simulink model "Feedback_2"  (R2017b)
settings: Solver=FixedStepDiscrete  StartTime=0.0  StopTime=10.0  FixedStep=.0001  RelTol=1e-3  EnableMultiTasking=on
libraries: stellaris_lp_lib x12, simulink x1
settings Model: Creator=Mitchell Cassaday  LastModifiedBy=Mitchell Cassaday
settings OptimizationCC: PassReuseOutputArgsAs=Individual arguments  MaxStackSize=64
settings DebuggingCC: ParameterTunabilityLossMsg=error
settings HardwareCC: ProdBitPerPointer=32  ProdBitPerSizeT=32  ProdBitPerPtrDiffT=32  ProdLargestAtomicInteger=Long  ProdLargestAtomicFloat=Double  ProdWordSize=32  ProdHWDeviceType=ARM Compatible->ARM Cortex
settings SFSimCC: MATLABDynamicMemAlloc=off
settings RTWCC: SystemTargetFile=ert.tlc  HardwareBoard=Tiva TM4C123G Launchpad  TLCOptions=-aInlineSetEventsForThisBaseRateFcn=TLC_FALSE -aSuppressMultiTaskScheduler=TLC_FALSE -aRateBasedStepFcn=1  TemplateMakefile=ert_default_tmf  GenerateReport=on  Toolchain=Texas Instruments Code Composer Studio (Tiva)  IncludeHyperlinkInReport=on  LaunchReport=on  GenerateTraceInfo=on  GenerateTraceReport=on  GenerateTraceReportSl=on  GenerateTraceReportSf=on  GenerateTraceReportEml=on
settings CodeAppCC: ForceParamTrailComments=on  IgnoreCustomStorageClasses=off  OperatorAnnotations=on  SimulinkDataObjDesc=on  SFDataObjDesc=on  InsertBlockDesc=on

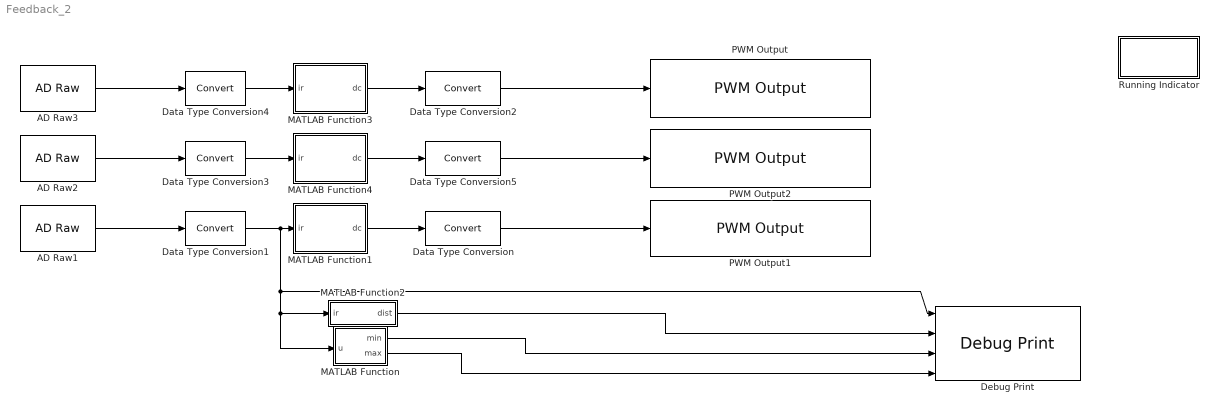
== system Feedback_2 ==
  AD Raw1 : stellaris_lp_lib/ADC/AD Raw  ch="2   PE2"  sample_time=.1
      settings: SourceProductName=Run on Stellaris LaunchPad
  AD Raw2 : stellaris_lp_lib/ADC/AD Raw  ch="3   PE1"  sample_time=.1
      settings: SourceProductName=Run on Stellaris LaunchPad
  AD Raw3 : stellaris_lp_lib/ADC/AD Raw  ch="5   PE5"  sample_time=.1
      settings: SourceProductName=Run on Stellaris LaunchPad
  Data Type Conversion{,1..5} (6 alike) : DataTypeConversion
  Debug Print : stellaris_lp_lib/Debug/Debug Print  fmt="'1:  %d    Dist  %d    min  %d    max  %d'"  sample_time=-1
      settings: SourceProductName=Run on Stellaris LaunchPad
  MATLAB Function : MATLAB Function  TreatAsAtomicUnit=on
  MATLAB Function1 : MATLAB Function  TreatAsAtomicUnit=on
  MATLAB Function2 : MATLAB Function  TreatAsAtomicUnit=on
  MATLAB Function3 : MATLAB Function  TreatAsAtomicUnit=on
  MATLAB Function4 : MATLAB Function  TreatAsAtomicUnit=on
  PWM Output : stellaris_lp_lib/PWM/PWM Output  ch="1    PC4"  invert=off  freq=1000  sample_time=-1
      settings: SourceProductName=Run on Stellaris LaunchPad
  PWM Output1 : stellaris_lp_lib/PWM/PWM Output  ch="3    PC6"  invert=off  freq=50000  sample_time=-1
      settings: SourceProductName=Run on Stellaris LaunchPad
  PWM Output2 : stellaris_lp_lib/PWM/PWM Output  ch="2    PC5"  invert=off  freq=1000  sample_time=-1
      settings: SourceProductName=Run on Stellaris LaunchPad
  Running Indicator : Subsystem
  wires:
  Data Type Conversion2/1 -> PWM Output/1
  Data Type Conversion/1 -> PWM Output1/1
  MATLAB Function1/1(dc) -> Data Type Conversion/1
  AD Raw1/1 -> Data Type Conversion1/1
  Data Type Conversion1/1 -> MATLAB Function/1(u), MATLAB Function2/1(ir), Debug Print/1, MATLAB Function1/1(ir)
  MATLAB Function/1(min) -> Debug Print/3
  MATLAB Function/2(max) -> Debug Print/4
  MATLAB Function2/1(dist) -> Debug Print/2
  AD Raw2/1 -> Data Type Conversion3/1
  AD Raw3/1 -> Data Type Conversion4/1
  Data Type Conversion4/1 -> MATLAB Function3/1(ir)
  MATLAB Function3/1(dc) -> Data Type Conversion2/1
  MATLAB Function4/1(dc) -> Data Type Conversion5/1
  Data Type Conversion5/1 -> PWM Output2/1
  Data Type Conversion3/1 -> MATLAB Function4/1(ir)

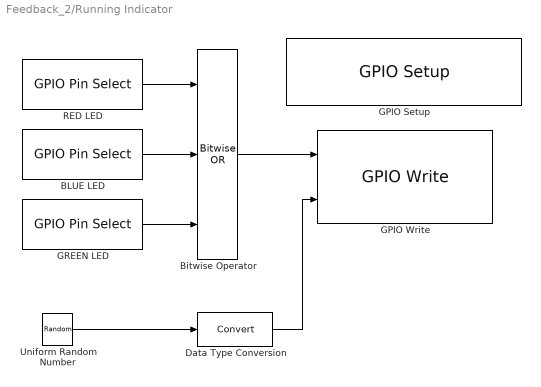
== system Feedback_2/Running Indicator ==
  BLUE LED : stellaris_lp_lib/GPIO/GPIO Pin Select  GPIO_PIN_X=GPIO_PIN_2
      settings: SourceProductName=Run on Stellaris LaunchPad
  Bitwise Operator : simulink/Logic and Bit Operations/Bitwise Operator  logicop=OR  UseBitMask=off  NumInputPorts=3  BitMask=bin2dec('11011001')  BitMaskRealWorld=Stored Integer
  Data Type Conversion : DataTypeConversion
  GPIO Setup : stellaris_lp_lib/GPIO/GPIO Setup  GPIO_PORTX_BASE=GPIO_PORTF_BASE  PinsOutput_0=Input  PinsOutput_1=Output  PinsOutput_2=Output  PinsOutput_3=Output  PinsOutput_4=Input  PinsOutput_5=Input  PinsOutput_6=Input  PinsOutput_7=Input
      settings: SourceProductName=Run on Stellaris LaunchPad
  GPIO Write : stellaris_lp_lib/GPIO/GPIO Write  GPIO_PORTX_BASE=GPIO_PORTF_BASE  SampleTime=-1
      settings: SourceProductName=Run on Stellaris LaunchPad
  GREEN LED : stellaris_lp_lib/GPIO/GPIO Pin Select  GPIO_PIN_X=GPIO_PIN_3
      settings: SourceProductName=Run on Stellaris LaunchPad
  RED LED : stellaris_lp_lib/GPIO/GPIO Pin Select  GPIO_PIN_X=GPIO_PIN_1
      settings: SourceProductName=Run on Stellaris LaunchPad
  Uniform Random Number : UniformRandomNumber  Minimum=2  Maximum=16  SampleTime=0.2
  wires:
  BLUE LED/1 -> Bitwise Operator/2
  RED LED/1 -> Bitwise Operator/1
  GREEN LED/1 -> Bitwise Operator/3
  Bitwise Operator/1 -> GPIO Write/1
  Uniform Random Number/1 -> Data Type Conversion/1
  Data Type Conversion/1 -> GPIO Write/2

== matlab function Feedback_2/MATLAB Function1 ==
  data: ir input; dc output
function dc = fcn(ir)
    min_ir = cast(220,'single');
    max_ir = cast(3860,'single');
    dc = cast(((cast(ir,'single')-min_ir) ./ (max_ir-min_ir) .* 100.0),'int32');

== matlab function Feedback_2/MATLAB Function ==
  data: u input; min output; max output
function [min,max] = fcn(u)
    persistent p_min;
    persistent p_max;
    
    if isempty(p_min)
        p_min = u;
        p_max = u;
        min = p_min;
        max = p_min;
    end
    
    if u < p_min
        min = u;
        p_min = u;
    else
        min = p_min;
    end
    if u > p_max
        max = u;
        p_max = u;
    else
        max = p_max;
    end

== matlab function Feedback_2/MATLAB Function2 ==
  data: ir input; dist output
function dist = fcn(ir)
    persistent ir_arr;
    persistent i;
    
    if isempty(ir_arr)
        ir_arr = zeros(20);
        for i = 1:20
            ir_arr(i) = ir;
        end
        i = 1;
    end
    ir_arr(i) = ir;
    avg = 0;
    for j = 1:20
        avg = avg + ir_arr(j);
    end
    avg = avg / 20;
    dist = cast(((avg - 230) / 5),'like',ir);
    
    if (i == 20)
        i = 0;
    end
    i = i + 1;
end

== matlab function Feedback_2/MATLAB Function3 ==
  data: ir input; dc output
function dc = fcn(ir)
    min_ir = cast(220,'single');
    max_ir = cast(3860,'single');
    dc = cast(((cast(ir,'single')-min_ir) ./ (max_ir-min_ir) .* 100.0),'int32');

== matlab function Feedback_2/MATLAB Function4 ==
  data: ir input; dc output
function dc = fcn(ir)
    min_ir = cast(220,'single');
    max_ir = cast(3860,'single');
    dc = cast(((cast(ir,'single')-min_ir) ./ (max_ir-min_ir) .* 100.0),'int32');
